simulink model "AMR_AutoModeControlUnit_24a"  (R2024a)
settings: configuration reference "SharedConfig" (kept outside this file)
undefined symbols (not defined in the file): gearbox_ratio, wheel_diameter
settings Model: DataDictionary=configuration_dictionary.sldd  Creator=matlab.cut  LastModifiedBy=matlab.cut
settings ConfigSetRef: SourceName=SharedConfig

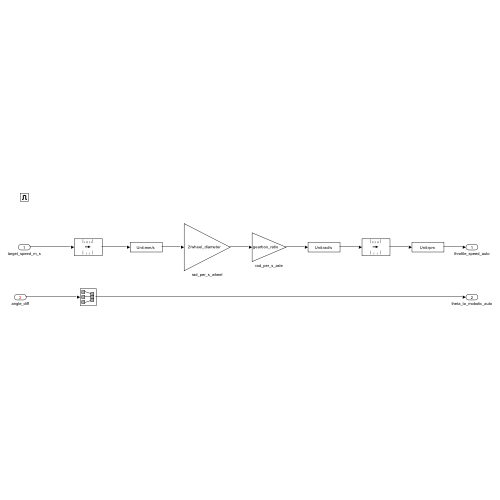
[thumbnail: Simulink's stored preview of the top-level diagram]
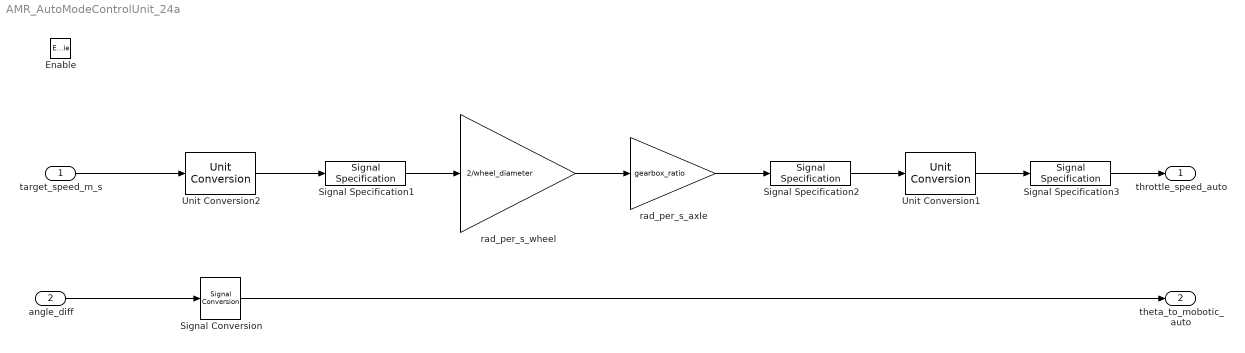
== system AMR_AutoModeControlUnit_24a ==
  target_speed_m_s : Inport  OutDataTypeStr=double  Unit=m/s  PortDimensions=1  SampleTime=[0.001,0]
  angle_diff : Inport  Port=2  OutDataTypeStr=double  PortDimensions=1  SampleTime=[0.001,0]
  Enable : EnablePort  SampleTime=[0.001,0]  OutDataTypeStr=boolean
  Signal Conversion : SignalConversion  OverrideOpt=off
  Signal Specification1 : SignalSpecification  Unit=mm/s
  Signal Specification2 : SignalSpecification  Unit=rad/s
  Signal Specification3 : SignalSpecification  Unit=rpm
  Unit Conversion1 : UnitConversion
  Unit Conversion2 : UnitConversion
  rad_per_s_axle : Gain  Gain=gearbox_ratio
  rad_per_s_wheel : Gain  Gain=2/wheel_diameter
  throttle_speed_auto : Outport  OutDataTypeStr=double  PortDimensions=1  SampleTime=[0.001,0]  OutputWhenDisabled=reset  InitialOutput=[0]
  theta_to_mobotic_auto : Outport  Port=2  OutDataTypeStr=double  PortDimensions=1  SampleTime=[0.001,0]  OutputWhenDisabled=reset  InitialOutput=[0]
  wires:
  angle_diff/1 -> Signal Conversion/1
  target_speed_m_s/1 -> Unit Conversion2/1
  Signal Specification2/1 -> Unit Conversion1/1
  Unit Conversion1/1 -> Signal Specification3/1
  Signal Specification3/1 -> throttle_speed_auto/1
  rad_per_s_wheel/1 -> rad_per_s_axle/1
  rad_per_s_axle/1 -> Signal Specification2/1
  Unit Conversion2/1 -> Signal Specification1/1
  Signal Specification1/1 -> rad_per_s_wheel/1
  Signal Conversion/1 -> theta_to_mobotic_auto/1
